simulink library "newPlant_cl"  (R2018b)
settings: Solver=VariableStepAuto  StartTime=0.0  StopTime=10.0  RelTol=1e-3
undefined symbols (not defined in the file): unstretched_l, X0
libraries: ayazGroundStation_cl x1, ayazLiftingBody_cl x1, ayazTethers_cl x1, ayazWinches_cl x1
settings Model: Creator=mcobb  LastModifiedBy=mcobb

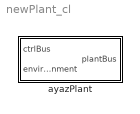
== system newPlant_cl ==
  ayazPlant : Subsystem

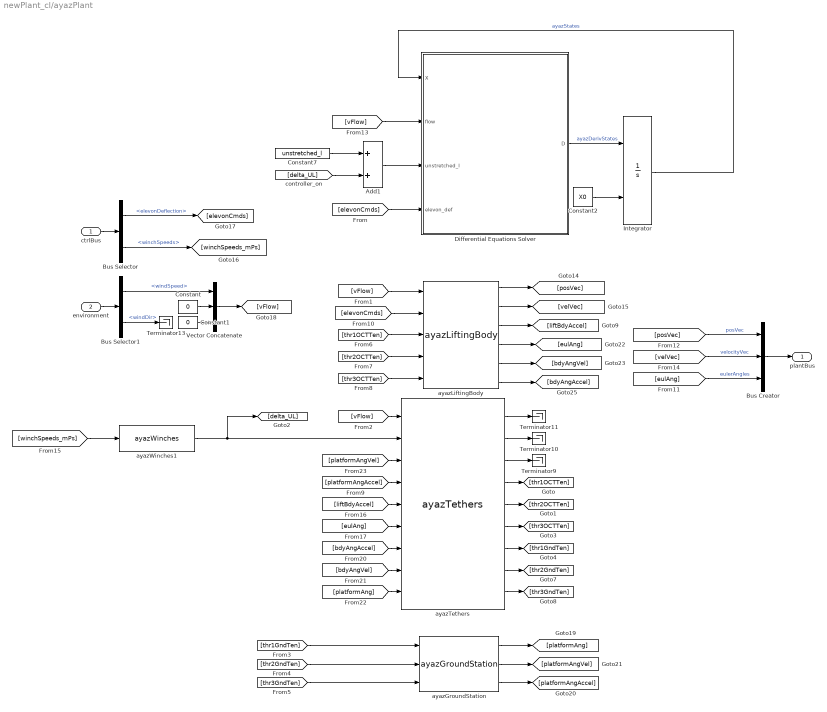
== system newPlant_cl/ayazPlant ==
  ctrlBus : Inport  OutDataTypeStr=Bus: ctrlBus
  environment : Inport  Port=2  OutDataTypeStr=Bus: envBus
  Add1 : Sum
  Bus Creator : BusCreator  Inputs=3  OutDataTypeStr=Bus: plantBus
  Bus Selector : BusSelector  OutputSignals=elevonDeflection,winchSpeeds
  Bus Selector1 : BusSelector  OutputSignals=windSpeed,windDir
  Constant : Constant  Value=0
  Constant1 : Constant  Value=0
  Constant2 : Constant  Value=X0
  Constant7 : Constant  Value=unstretched_l
  Differential Equations Solver : MATLAB Function  TreatAsAtomicUnit=on
  Integrator : Integrator  InitialConditionSource=external  InitialCondition=X0
  Terminator{9..11,13} (4 alike) : Terminator
  Vector Concatenate : Concatenate  NumInputs=3
  ayazGroundStation : ayazGroundStation_cl/ayazGroundStation  SystemSampleTime=-1
  ayazLiftingBody : ayazLiftingBody_cl/ayazLiftingBody  SystemSampleTime=-1
  ayazTethers : ayazTethers_cl/ayazTethers  SystemSampleTime=-1
  ayazWinches1 : ayazWinches_cl/ayazWinches  SystemSampleTime=-1
  plantBus : Outport  OutDataTypeStr=Bus: plantBus
  wires:
  Constant7/1 -> Add1/1
  Add1/1 -> Differential Equations Solver/3(unstretched_l)
  [elevonCmds] -> Differential Equations Solver/4(elevon_def)
  [delta_UL] -> Add1/2
  Constant2/1 -> Integrator/2
  Integrator/1 -> Differential Equations Solver/1(X)  "ayazStates"
  Differential Equations Solver/1(D) -> Integrator/1  "ayazDerivStates"
  ayazTethers/4 -> [thr1OCTTen]
  ayazTethers/6 -> [thr3OCTTen]
  ayazTethers/5 -> [thr2OCTTen]
  ayazTethers/7 -> [thr1GndTen]
  ayazTethers/8 -> [thr2GndTen]
  ayazTethers/9 -> [thr3GndTen]
  ayazTethers/3 -> Terminator9/1
  ayazTethers/2 -> Terminator10/1
  ayazTethers/1 -> Terminator11/1
  ayazWinches1/1 -> [delta_UL], ayazTethers/2
  ayazLiftingBody/3 -> [liftBdyAccel]
  ayazLiftingBody/4 -> [eulAng]
  ayazLiftingBody/1 -> [posVec]
  ayazLiftingBody/2 -> [velVec]
  [vFlow] -> ayazTethers/1
  [vFlow] -> ayazLiftingBody/1
  [thr1GndTen] -> ayazGroundStation/1
  [thr2GndTen] -> ayazGroundStation/2
  [thr3GndTen] -> ayazGroundStation/3
  [thr1OCTTen] -> ayazLiftingBody/3
  [thr2OCTTen] -> ayazLiftingBody/4
  [thr3OCTTen] -> ayazLiftingBody/5
  [winchSpeeds_mPs] -> ayazWinches1/1
  [elevonCmds] -> ayazLiftingBody/2
  environment/1 -> Bus Selector1/1
  ctrlBus/1 -> Bus Selector/1
  Bus Selector1/2 -> Terminator13/1  "<windDir>"
  Bus Selector/1 -> [elevonCmds]  "<elevonDeflection>"
  Bus Selector1/1 -> Vector Concatenate/1  "<windSpeed>"
  Bus Selector/2 -> [winchSpeeds_mPs]  "<winchSpeeds>"
  Bus Creator/1 -> plantBus/1
  [posVec] -> Bus Creator/1  "posVec"
  [eulAng] -> Bus Creator/3  "eulerAngles"
  [velVec] -> Bus Creator/2  "velocityVec"
  Vector Concatenate/1 -> [vFlow]
  Constant/1 -> Vector Concatenate/2
  Constant1/1 -> Vector Concatenate/3
  ayazGroundStation/1 -> [platformAng]
  ayazGroundStation/2 -> [platformAngVel]
  [platformAngAccel] -> ayazTethers/4
  [liftBdyAccel] -> ayazTethers/5
  [eulAng] -> ayazTethers/6
  [bdyAngAccel] -> ayazTethers/7
  [bdyAngVel] -> ayazTethers/8
  [platformAng] -> ayazTethers/9
  [platformAngVel] -> ayazTethers/3
  ayazGroundStation/3 -> [platformAngAccel]
  ayazLiftingBody/5 -> [bdyAngVel]
  ayazLiftingBody/6 -> [bdyAngAccel]
  [vFlow] -> Differential Equations Solver/2(flow)

== matlab function newPlant_cl/ayazPlant/Differential Equations Solver ==
  data: X input; D output; flow input; unstretched_l input; elevon_def input; sim_param parameter
function D = multimode_ode(X,flow,unstretched_l,elevon_def,sim_param)

D = zeros(size(X));

% loader = load('sim_param.mat');
% 
% sim_param = loader.sim_param;

%% number of nodes
N = sim_param.N;

% extract other values
mass = sim_param.geom_param.mass;
MI = sim_param.geom_param.MI;

P_Izz = sim_param.platform_param.platform_Izz;
cp = sim_param.platform_param.platform_damping;

R1n_cm = sim_param.tether_imp_nodes.R1n_cm;
R2n_cm = sim_param.tether_imp_nodes.R2n_cm;
R3n_cm = sim_param.tether_imp_nodes.R3n_cm;

R11_g = sim_param.tether_imp_nodes.R11_g;
R21_g = sim_param.tether_imp_nodes.R21_g;
R31_g = sim_param.tether_imp_nodes.R31_g;


%% constants
m = mass;
Ixx = MI(1,1);
Iyy = MI(2,2);
Izz = MI(3,3);

m_added = sim_param.geom_param.m_added;
Izz_added = sim_param.geom_param.Izz_added;

%% extract values from state space
% lifting body values
Rcm_o = X(1:3,1);
O_Vcm_o = X(4:6,1);

euler_ang = X(7:9,1);
ph = euler_ang(1);
th = euler_ang(2);
ps = euler_ang(3);

% rotations
[oCb,bCo] = rotation_sequence(euler_ang);

OwB = X(10:12,1);
wx = OwB(1);
wy = OwB(2);
wz = OwB(3);

psi_p = X(13,1);
platform_ang_vel = X(14,1);

pCo = [cos(psi_p) sin(psi_p) 0; -sin(psi_p) cos(psi_p) 0; 0 0 1];
oCp = pCo';


% tether position and velocity components
R1i_o = X(15:(14 + 3*N),1);
R2i_o = X((15 + 3*N):(14 + 6*N),1);
R3i_o = X((15 + 6*N):(14 + 9*N),1);

O_V1i_o = X((15 + 9*N):(14 + 12*N),1);
O_V2i_o = X((15 + 12*N):(14 + 15*N),1);
O_V3i_o = X((15 + 15*N):(14 + 18*N),1);


%%  center of mass first derivatives
D(1:3,1) = O_Vcm_o;
D(7,1) = wx + sin(ph)*tan(th)*wy + cos(ph)*tan(th)*wz;
D(8,1) = cos(ph)*wy - sin(ph)*wz;
D(9,1) = sec(th)*sin(ph)*wy + cos(ph)*sec(th)*wz;

%% platofrm angle first derivates
D(13,1) = platform_ang_vel;
OwP = [0;0;platform_ang_vel];

%% grnd station first derivative
D(15:17,1) = [0;0;0];

%% changing first node first deivative
O_V1i_o(1:3,1) = oCp*(cross(OwP,R11_g));
O_V2i_o(1:3,1) = oCp*(cross(OwP,R21_g));
O_V3i_o(1:3,1) = oCp*(cross(OwP,R31_g));

%% changing last node first deivative
O_V1i_o((end-2):end,1) = O_Vcm_o + oCb*(cross(OwB,R1n_cm));
O_V2i_o((end-2):end,1)=  O_Vcm_o + oCb*(cross(OwB,R2n_cm));
O_V3i_o((end-2):end,1)=  O_Vcm_o + oCb*(cross(OwB,R3n_cm));

%% tether nodes first derivatives
D(15:(14 + 3*N),1) = O_V1i_o;
D((15 + 3*N):(14 + 6*N),1) = O_V2i_o;
D((15 + 6*N):(14 + 9*N),1) = O_V3i_o;


%% EXTERNAL FORCES AND TORQUES
op = multinode_F_and_T_external(sim_param,flow,unstretched_l,elevon_def,Rcm_o,R1i_o,R2i_o,R3i_o,...
    O_Vcm_o,O_V1i_o,O_V2i_o,O_V3i_o,OwB,euler_ang,psi_p);

O_F_ext = op.O_F_ext;
B_T_ext = op.B_T_ext;
sum_1_f = op.sum_1_f;
sum_2_f = op.sum_2_f;
sum_3_f = op.sum_3_f;
T_o_ext = op.T_o_ext;

Tx = B_T_ext(1);
Ty = B_T_ext(2);
Tz = B_T_ext(3);

% mass at each node
tether_masses = op.tether_masses;

m1i = tether_masses(1)/N;
m2i = tether_masses(2)/N;
m3i = tether_masses(3)/N;

%% center of mass second derivatives
% added mass
mass_matrix = [1/(m+m_added(1)) 0 0;0 1/(m+m_added(2)) 0;0 0 1/(m+m_added(3))];

D(4:6,1) = oCb*(mass_matrix*(bCo*O_F_ext));
D(10,1) = (1/Ixx)*(Tx + (Iyy - Izz)*wy*wz);
D(11,1) = (1/Iyy)*(Ty + (Izz - Ixx)*wx*wz);
D(12,1) = (1/(Izz+Izz_added))*(Tz + (Ixx - Iyy)*wx*wy);

OaB = D(10:12,1);

%% platform angle second derivative
D(14,1) = (T_o_ext/P_Izz) - cp*platform_ang_vel;
OaP = [0;0;D(14,1)];

%% tether nodes 2nd derivatives

for i = 1:N
    
    if i == 1
        D((14 + 9*N + 3*i - 2):(14 + 9*N + 3*i),1) = oCp*( cross(OaP,R11_g) +  cross(OwP,(cross(OwP,R11_g))) );
        D((14 + 12*N + 3*i - 2):(14 + 12*N + 3*i),1) = oCp*( cross(OaP,R21_g) +  cross(OwP,(cross(OwP,R21_g))) );
        D((14 + 15*N + 3*i - 2):(14 + 15*N + 3*i),1) = oCp*( cross(OaP,R31_g) +  cross(OwP,(cross(OwP,R31_g))) );
        
    elseif i>1 && i<N
        
        D((14 + 9*N + 3*i - 2):(14 + 9*N + 3*i),1) = (1/m1i)*sum_1_f(:,i);
        D((14 + 12*N + 3*i - 2):(14 + 12*N + 3*i),1) = (1/m2i)*sum_2_f(:,i);
        D((14 + 15*N + 3*i - 2):(14 + 15*N + 3*i),1) = (1/m3i)*sum_3_f(:,i);
        
    elseif i == N
        
        D((14 + 9*N + 3*i - 2):(14 + 9*N + 3*i),1) = D(4:6,1) + ...
            oCb*( cross(OaB,R1n_cm) +  cross(OwB,(cross(OwB,R1n_cm))) );
        
        
        D((14 + 12*N + 3*i - 2):(14 + 12*N + 3*i),1) =  D(4:6,1) + ...
            oCb*( cross(OaB,R2n_cm) +  cross(OwB,(cross(OwB,R2n_cm))) ) ;
        
        D((14 + 15*N + 3*i - 2):(14 + 15*N + 3*i),1) =  D(4:6,1) + ...
            oCb*( cross(OaB,R3n_cm) +  cross(OwB,(cross(OwB,R3n_cm))) );
        
    end
    
    
end
% x = 1;

end
